simulink model "FOSimplified"  (R2015b)
settings: Solver=ode45  StartTime=0.0  StopTime=100  RelTol=1e-3
libraries: simulink x1
settings Model: Creator=Administrator  LastModifiedBy=Administrator
settings DataIOCC: LimitDataPoints=off

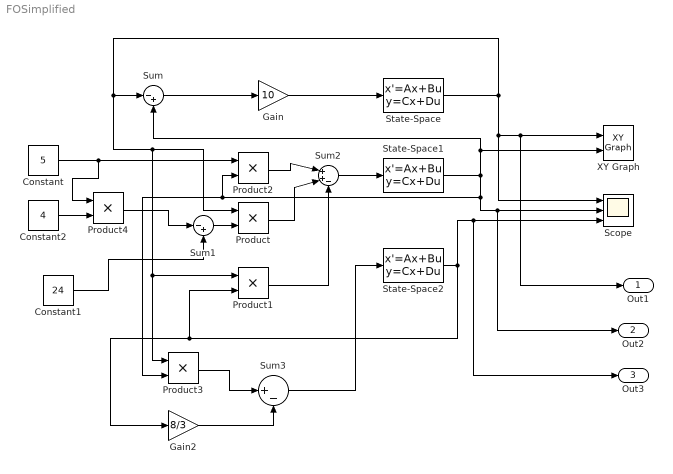
== system FOSimplified ==
  Constant : Constant  Value=5
  Constant1 : Constant  Value=24
  Constant2 : Constant  Value=4
  Gain : Gain  Gain=10
  Gain2 : Gain  Gain=8/3
  Product{,1..4} (5 alike) : Product
  Scope : Scope  NumInputPorts=3
  State-Space : StateSpace  A=[-1423, -16.0087;1,0]  B=[1,0]'  C=[1.2974, 1459.6]  D=0  X0=1
  State-Space1 : StateSpace  A=[-1423, -16.0087;1,0]  B=[1,0]'  C=[1.2974, 1459.6]  D=0  X0=1
  State-Space2 : StateSpace  A=[-1423, -16.0087;1,0]  B=[1,0]'  C=[1.2974, 1459.6]  D=0  X0=1
  Sum : Sum  Inputs=|-+
  Sum1 : Sum  Inputs=|-+
  Sum2 : Sum  Inputs=|++-
  Sum3 : Sum  Inputs=|+-
  XY Graph : simulink/Sinks/XY Graph  xmin=-40  xmax=40  ymin=-40  ymax=40  st=-1
  Out1 : Outport
  Out2 : Outport  Port=2
  Out3 : Outport  Port=3
  wires:
  Gain/1 -> State-Space/1
  State-Space/1 -> Scope/1, Out1/1, XY Graph/1, Sum/1, Product3/1, Product1/1, Product/1
  Sum/1 -> Gain/1
  State-Space1/1 -> Product2/2, Product3/2, Out2/1, Scope/2, XY Graph/2, Sum/2
  Constant/1 -> Product4/1, Product2/1
  Product4/1 -> Sum1/1
  Constant1/1 -> Sum1/2
  Sum1/1 -> Product/2
  State-Space2/1 -> Gain2/1, Product1/2, Out3/1, Scope/3
  Product1/1 -> Sum2/3
  Product2/1 -> Sum2/1
  Product/1 -> Sum2/2
  Sum2/1 -> State-Space1/1
  Product3/1 -> Sum3/1
  Gain2/1 -> Sum3/2
  Sum3/1 -> State-Space2/1
  Constant2/1 -> Product4/2
